simulink model "hnn"  (R2024b)
settings: Solver=VariableStepAuto  StartTime=0.0  StopTime=10.0  RelTol=1e-3
settings Model: Creator=merlin  LastModifiedBy=merlin

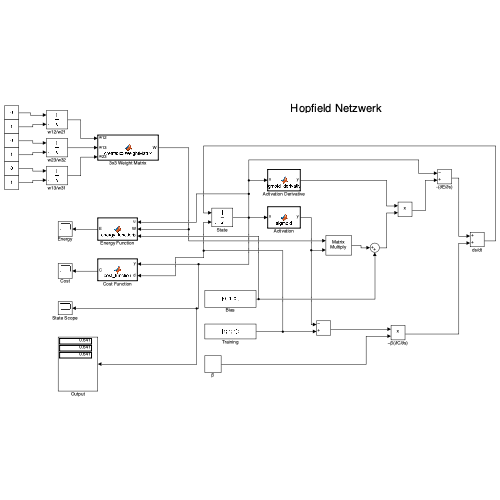
[thumbnail: Simulink's stored preview of the top-level diagram]
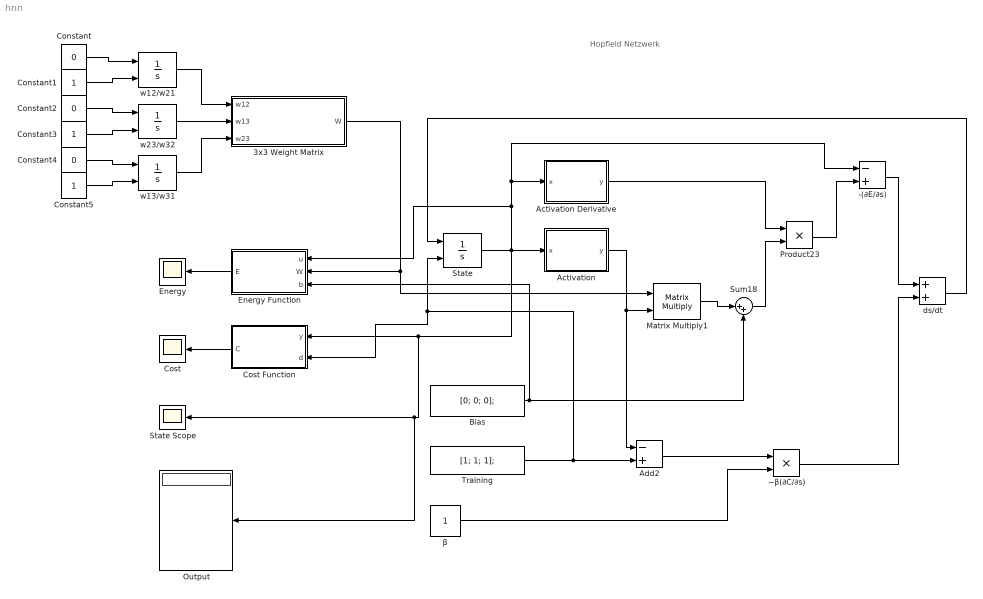
== system hnn ==
  note: Hopfield Netzwerk
  -(∂E/∂s) : Sum  Inputs=-+
  3x3 Weight Matrix : MATLAB Function  TreatAsAtomicUnit=on
  Activation : MATLAB Function  TreatAsAtomicUnit=on
  Activation Derivative : MATLAB Function  TreatAsAtomicUnit=on
  Add2 : Sum  Inputs=-+
  Bias : Constant  Value=[0; 0; 0];  VectorParams1D=off
  Constant : Constant  Value=0
  Constant1 : Constant
  Constant2 : Constant  Value=0
  Constant3 : Constant
  Constant4 : Constant  Value=0
  Constant5 : Constant
  Cost : Scope
  Cost Function : MATLAB Function  TreatAsAtomicUnit=on
  Energy : Scope
  Energy Function : MATLAB Function  TreatAsAtomicUnit=on
  Matrix Multiply1 : Product  Multiplication=Matrix(*)
  Output : Display
  Product23 : Product
  State : Integrator  InitialConditionSource=external
  State Scope : Scope
  Sum18 : Sum  Inputs=|++
  Training : Constant  Value=[1; 1; 1];  VectorParams1D=off
  ds/dt : Sum
  w12/w21 : Integrator  InitialConditionSource=external
  w13/w31 : Integrator  InitialConditionSource=external
  w23/w32 : Integrator  InitialConditionSource=external
  β : Constant  VectorParams1D=off
  −β(∂C/∂s) : Product
  wires:
  w12/w21/1 -> 3x3 Weight Matrix/1(w12)
  w23/w32/1 -> 3x3 Weight Matrix/2(w13)
  w13/w31/1 -> 3x3 Weight Matrix/3(w23)
  Constant/1 -> w12/w21/1
  Constant1/1 -> w12/w21/2
  Constant2/1 -> w23/w32/1
  Constant3/1 -> w23/w32/2
  Constant4/1 -> w13/w31/1
  Constant5/1 -> w13/w31/2
  Bias/1 -> Sum18/2, Energy Function/3(b)
  ds/dt/1 -> State/1
  Energy Function/1(E) -> Energy/1
  State/1 -> Cost Function/1(y), Output/1, State Scope/1, Activation Derivative/1(x), -(∂E/∂s)/1, Energy Function/1(u), Activation/1(x)
  β/1 -> −β(∂C/∂s)/2
  Training/1 -> Cost Function/2(d), State/2, Add2/2
  Activation/1(y) -> Add2/1, Matrix Multiply1/2
  -(∂E/∂s)/1 -> ds/dt/1
  Add2/1 -> −β(∂C/∂s)/1
  Matrix Multiply1/1 -> Sum18/1
  Activation Derivative/1(y) -> Product23/1
  Sum18/1 -> Product23/2
  −β(∂C/∂s)/1 -> ds/dt/2
  Cost Function/1(C) -> Cost/1
  Product23/1 -> -(∂E/∂s)/2
  3x3 Weight Matrix/1(W) -> Energy Function/2(W), Matrix Multiply1/1

== matlab function hnn/3x3 Weight Matrix ==
  data: w12 input; W output; w13 input; w23 input
function W = create3x3WeightMatrix(w12, w13, w23)
    W = [0,    w12,  w13;
         w12,  0,    w23;
         w13,  w23,  0];
end

== matlab function hnn/Energy Function ==
  data: u input; E output; W input; b input
function E = energy_function(u, W, b)
    rho = @(x) 1 ./ (1 + exp(-x));

    E = (1/2) * sum(u.^2) ...
        - (1/2) * sum(sum(W .* (rho(u) * rho(u)')))
        - sum(b .* rho(u));
end

== matlab function hnn/Activation Derivative ==
  data: x input; y output
function y = sigmoid_derivative(x)
sigmoid = 1 ./ (1 + exp(-x));
y = sigmoid .* (1 - sigmoid);
end

== matlab function hnn/Activation ==
  data: x input; y output
function y = sigmoid(x)
y = 1 ./ (1 + exp(-x));
end

== matlab function hnn/Cost Function ==
  data: y input; C output; d input
function C = cost_function(y, d)
    C = 0.5 * sum((y - d).^2);
end
